simulink model "Complementary_filter_simulink"  (R2022b)
settings: Solver=FixedStepAuto  StartTime=0.0  StopTime=90.0  FixedStep=0.01  RelTol=1e-3
undefined symbols (not defined in the file or in its folder): DiscIntNeverNeededParam
settings Model: Creator=mosta  LastModifiedBy=mosta

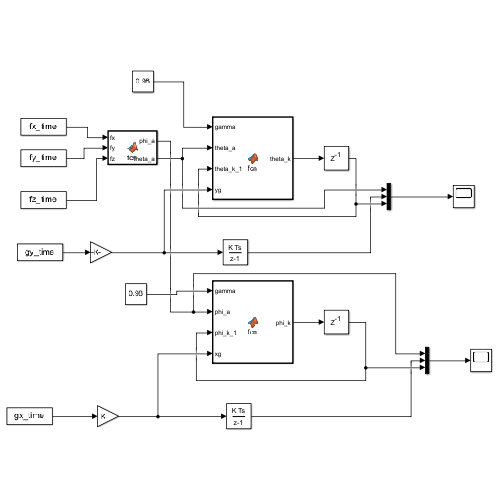
[thumbnail: Simulink's stored preview of the top-level diagram]
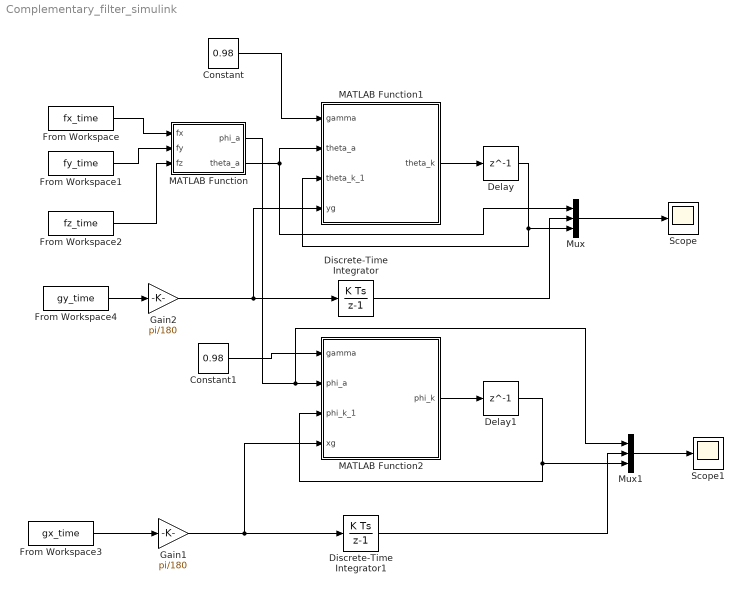
== system Complementary_filter_simulink ==
  Constant : Constant  Value=0.98
  Constant1 : Constant  Value=0.98
  Delay : Delay  DelayLength=1
  Delay1 : Delay  DelayLength=1
  Discrete-Time Integrator : DiscreteIntegrator  SampleTime=-1  ICPrevOutput=DiscIntNeverNeededParam  ICPrevScaledInput=DiscIntNeverNeededParam
  Discrete-Time Integrator1 : DiscreteIntegrator  SampleTime=-1  ICPrevOutput=DiscIntNeverNeededParam  ICPrevScaledInput=DiscIntNeverNeededParam
  From Workspace : FromWorkspace  VariableName=fx_time
  From Workspace1 : FromWorkspace  VariableName=fy_time
  From Workspace2 : FromWorkspace  VariableName=fz_time
  From Workspace3 : FromWorkspace  VariableName=gx_time
  From Workspace4 : FromWorkspace  VariableName=gy_time
  Gain1 : Gain  Gain=pi/180
  Gain2 : Gain  Gain=pi/180
  MATLAB Function : MATLAB Function  TreatAsAtomicUnit=on
  MATLAB Function1 : MATLAB Function  TreatAsAtomicUnit=on
  MATLAB Function2 : MATLAB Function  TreatAsAtomicUnit=on
  Mux : Mux  Inputs=3
  Mux1 : Mux  Inputs=3
  Scope : Scope
  Scope1 : Scope
  wires:
  From Workspace4/1 -> Gain2/1
  Gain2/1 -> Discrete-Time Integrator/1, MATLAB Function1/4(yg)
  From Workspace/1 -> MATLAB Function/1(fx)
  From Workspace1/1 -> MATLAB Function/2(fy)
  From Workspace2/1 -> MATLAB Function/3(fz)
  MATLAB Function/2(theta_a) -> MATLAB Function1/2(theta_a), Mux/1
  Constant/1 -> MATLAB Function1/1(gamma)
  Delay/1 -> Mux/3, MATLAB Function1/3(theta_k_1)
  MATLAB Function1/1(theta_k) -> Delay/1
  Discrete-Time Integrator/1 -> Mux/2
  Mux/1 -> Scope/1
  Constant1/1 -> MATLAB Function2/1(gamma)
  From Workspace3/1 -> Gain1/1
  Gain1/1 -> Discrete-Time Integrator1/1, MATLAB Function2/4(xg)
  MATLAB Function/1(phi_a) -> Mux1/1, MATLAB Function2/2(phi_a)
  MATLAB Function2/1(phi_k) -> Delay1/1
  Delay1/1 -> Mux1/3, MATLAB Function2/3(phi_k_1)
  Discrete-Time Integrator1/1 -> Mux1/2
  Mux1/1 -> Scope1/1

== matlab function Complementary_filter_simulink/MATLAB Function1 ==
  data: gamma input; theta_k output; theta_a input; theta_k_1 input; yg input
function theta_k = fcn(gamma, theta_a,theta_k_1,yg)

theta_k = (1-gamma)*theta_a+gamma*(theta_k_1+0.01*yg);
end

== matlab function Complementary_filter_simulink/MATLAB Function ==
  data: phi_a output; fx input; theta_a output; fy input; fz input
function [phi_a,theta_a] = fcn(fx,fy,fz)
    phi_a = atan2(fy,fz);
    theta_a = atan2(-fx,sqrt(fy.^2+fz.^2));
end

== matlab function Complementary_filter_simulink/MATLAB Function2 ==
  data: gamma input; phi_k output; phi_a input; phi_k_1 input; xg input
function phi_k = fcn(gamma, phi_a,phi_k_1,xg)

phi_k = (1-gamma)*phi_a+gamma*(phi_k_1+0.01*xg);
end
